simulink model "IEEE14_case"  (R2024b)
settings: Solver=FixedStepAuto  StartTime=0  StopTime=2  FixedStep=1e-7  RelTol=1e-3
values from neighbouring files (symbols this model uses):
  GFL_15_Bva = 0.009    [IEEE14_parameters.m]
  GFL_15_C_bus_pu = 7.179419    [IEEE14_parameters.m]
  GFL_15_f0 = 60    [IEEE14_parameters.m]
  GFL_15_I_id = 691.26967    [IEEE14_parameters.m]
  GFL_15_I_iq = 691.26967    [IEEE14_parameters.m]
  GFL_15_I_od = 45.2207    [IEEE14_parameters.m]
  GFL_15_I_oq = 45.2207    [IEEE14_parameters.m]
  GFL_15_I_pll = 0.78    [IEEE14_parameters.m]
  GFL_15_Kdi = 0.09    [IEEE14_parameters.m]
  GFL_15_Kdo = 0.9    [IEEE14_parameters.m]
  GFL_15_Kqi = 0.09    [IEEE14_parameters.m]
  GFL_15_Kqo = 0.9    [IEEE14_parameters.m]
  GFL_15_Lg_pu = 0.631447    [IEEE14_parameters.m]
  GFL_15_mode = 1    [IEEE14_parameters.m]
  GFL_15_P_id = 3.7166    [IEEE14_parameters.m]
  GFL_15_P_iq = 3.7166    [IEEE14_parameters.m]
  GFL_15_P_od = 0.4798    [IEEE14_parameters.m]
  GFL_15_P_oq = 0.4798    [IEEE14_parameters.m]
  GFL_15_P_pll = 290.42    [IEEE14_parameters.m]
  GFL_15_Qe_ref = 0.2    [IEEE14_parameters.m]
  GFL_15_Rg_pu = 0.024016    [IEEE14_parameters.m]
  GFL_15_Sbase = 1.000000e+4    (= 10000)    [IEEE14_parameters.m]
  GFL_15_Tdi = 0.01    [IEEE14_parameters.m]
  GFL_15_Tdo = 0.2    [IEEE14_parameters.m]
  GFL_15_Tqi = 0.01    [IEEE14_parameters.m]
  GFL_15_Tqo = 0.2    [IEEE14_parameters.m]
  GFL_15_Vbase = 380    [IEEE14_parameters.m]
  GFL_15_Vdc_ref = 1.011475    [IEEE14_parameters.m]
  GFL_15_Vdcbase = 700    [IEEE14_parameters.m]
  GFL_15_vq_ref = 0    [IEEE14_parameters.m]
  GFL_16_Bva = 0.002    [IEEE14_parameters.m]
  GFL_16_C_bus_pu = 7.179419    [IEEE14_parameters.m]
  GFL_16_f0 = 60    [IEEE14_parameters.m]
  GFL_16_I_id = 691.26967    [IEEE14_parameters.m]
  GFL_16_I_iq = 691.26967    [IEEE14_parameters.m]
  GFL_16_I_od = 45.2207    [IEEE14_parameters.m]
  GFL_16_I_oq = 45.2207    [IEEE14_parameters.m]
  GFL_16_I_pll = 0.78    [IEEE14_parameters.m]
  GFL_16_Kdi = 0.05    [IEEE14_parameters.m]
  GFL_16_Kdo = 0.5    [IEEE14_parameters.m]
  GFL_16_Kqi = 0.05    [IEEE14_parameters.m]
  GFL_16_Kqo = 0.5    [IEEE14_parameters.m]
  GFL_16_Lg_pu = 0.631447    [IEEE14_parameters.m]
  GFL_16_mode = 1    [IEEE14_parameters.m]
  GFL_16_P_id = 3.7166    [IEEE14_parameters.m]
  GFL_16_P_iq = 3.7166    [IEEE14_parameters.m]
  GFL_16_P_od = 0.4798    [IEEE14_parameters.m]
  GFL_16_P_oq = 0.4798    [IEEE14_parameters.m]
  GFL_16_P_pll = 290.42    [IEEE14_parameters.m]
  GFL_16_Qe_ref = 0.2    [IEEE14_parameters.m]
  GFL_16_Rg_pu = 0.024016    [IEEE14_parameters.m]
  GFL_16_Sbase = 1.000000e+4    (= 10000)    [IEEE14_parameters.m]
  GFL_16_Tdi = 0.01    [IEEE14_parameters.m]
  GFL_16_Tdo = 0.2    [IEEE14_parameters.m]
  GFL_16_Tqi = 0.01    [IEEE14_parameters.m]
  GFL_16_Tqo = 0.2    [IEEE14_parameters.m]
  GFL_16_Vbase = 380    [IEEE14_parameters.m]
  GFL_16_Vdc_ref = 1.01144    [IEEE14_parameters.m]
  GFL_16_Vdcbase = 700    [IEEE14_parameters.m]
  GFL_16_vq_ref = 0    [IEEE14_parameters.m]
  GFL_17_Bva = 0.002    [IEEE14_parameters.m]
  GFL_17_C_bus_pu = 7.179419    [IEEE14_parameters.m]
  GFL_17_f0 = 60    [IEEE14_parameters.m]
  GFL_17_I_id = 691.26967    [IEEE14_parameters.m]
  GFL_17_I_iq = 691.26967    [IEEE14_parameters.m]
  GFL_17_I_od = 45.2207    [IEEE14_parameters.m]
  GFL_17_I_oq = 45.2207    [IEEE14_parameters.m]
  GFL_17_I_pll = 0.78    [IEEE14_parameters.m]
  GFL_17_Kdi = 0.05    [IEEE14_parameters.m]
  GFL_17_Kdo = 0.5    [IEEE14_parameters.m]
  GFL_17_Kqi = 0.05    [IEEE14_parameters.m]
  GFL_17_Kqo = 0.5    [IEEE14_parameters.m]
  GFL_17_Lg_pu = 0.631447    [IEEE14_parameters.m]
  GFL_17_mode = 1    [IEEE14_parameters.m]
  GFL_17_P_id = 3.7166    [IEEE14_parameters.m]
  GFL_17_P_iq = 3.7166    [IEEE14_parameters.m]
  GFL_17_P_od = 0.4798    [IEEE14_parameters.m]
  GFL_17_P_oq = 0.4798    [IEEE14_parameters.m]
  GFL_17_P_pll = 290.42    [IEEE14_parameters.m]
  GFL_17_Qe_ref = 0.2    [IEEE14_parameters.m]
  GFL_17_Rg_pu = 0.024016    [IEEE14_parameters.m]
  GFL_17_Sbase = 1.000000e+4    (= 10000)    [IEEE14_parameters.m]
  GFL_17_Tdi = 0.01    [IEEE14_parameters.m]
  GFL_17_Tdo = 0.2    [IEEE14_parameters.m]
  GFL_17_Tqi = 0.01    [IEEE14_parameters.m]
  GFL_17_Tqo = 0.2    [IEEE14_parameters.m]
  GFL_17_Vbase = 380    [IEEE14_parameters.m]
  GFL_17_Vdc_ref = 1.011632    [IEEE14_parameters.m]
  GFL_17_Vdcbase = 700    [IEEE14_parameters.m]
  GFL_17_vq_ref = 0    [IEEE14_parameters.m]
  GFL_18_Bva = 0.002    [IEEE14_parameters.m]
  GFL_18_C_bus_pu = 7.179419    [IEEE14_parameters.m]
  GFL_18_f0 = 60    [IEEE14_parameters.m]
  GFL_18_I_id = 691.26967    [IEEE14_parameters.m]
  GFL_18_I_iq = 691.26967    [IEEE14_parameters.m]
  GFL_18_I_od = 45.2207    [IEEE14_parameters.m]
  GFL_18_I_oq = 45.2207    [IEEE14_parameters.m]
  GFL_18_I_pll = 0.78    [IEEE14_parameters.m]
  GFL_18_Kdi = 0.05    [IEEE14_parameters.m]
  GFL_18_Kdo = 0.5    [IEEE14_parameters.m]
  GFL_18_Kqi = 0.05    [IEEE14_parameters.m]
  GFL_18_Kqo = 0.5    [IEEE14_parameters.m]
  GFL_18_Lg_pu = 0.631447    [IEEE14_parameters.m]
  GFL_18_mode = 1    [IEEE14_parameters.m]
  GFL_18_P_id = 3.7166    [IEEE14_parameters.m]
  GFL_18_P_iq = 3.7166    [IEEE14_parameters.m]
  GFL_18_P_od = 0.4798    [IEEE14_parameters.m]
  GFL_18_P_oq = 0.4798    [IEEE14_parameters.m]
  GFL_18_P_pll = 290.42    [IEEE14_parameters.m]
  GFL_18_Qe_ref = 0.2    [IEEE14_parameters.m]
  GFL_18_Rg_pu = 0.024016    [IEEE14_parameters.m]
  GFL_18_Sbase = 1.000000e+4    (= 10000)    [IEEE14_parameters.m]
  GFL_18_Tdi = 0.01    [IEEE14_parameters.m]
  GFL_18_Tdo = 0.2    [IEEE14_parameters.m]
  GFL_18_Tqi = 0.01    [IEEE14_parameters.m]
  GFL_18_Tqo = 0.2    [IEEE14_parameters.m]
  GFL_18_Vbase = 380    [IEEE14_parameters.m]
  GFL_18_Vdc_ref = 1.011572    [IEEE14_parameters.m]
  GFL_18_Vdcbase = 700    [IEEE14_parameters.m]
  GFL_18_vq_ref = 0    [IEEE14_parameters.m]
  ... (+180 more)
(part 25 of 25)

== system IEEE14_case/SG_D_8/i_q_SG_D_8_block ==
  note: i_q_SG_D_8 in case14gfl
      | $-\frac{\sin\left(\theta _{\mathrm{SG},D,8}\right)\,\left(\psi _{q,\mathrm{SG},D,8}+\frac{\psi _{\mathrm{gq},\mathrm{SG},D,8}\,\left(x_{l}-x_{\mathrm{qdd}}\right)}{x_{l}-x_{\mathrm{qd}}}+\frac{\psi _{\mathrm{kq},\mathrm{SG},D,8}\,\left(x_{\mathrm{qd}}-x_{\mathrm{qdd}}\right)}{x_{l}-x_{\mathrm{qd}}}\right)}{x_{\mathrm{qdd}}}-\frac{\cos\left(\theta _{\mathrm{SG},D,8}\right)\,\left(\frac{\psi _{\mathrm{1d},\mathrm{SG},D,8}\,\left(x_{\mathrm{dd}}-x_{\mathrm{ddd}}\right)}{x_{\mathrm{dd}}-x_{l}}-\psi _{d,\mathrm{SG},D,8}+\frac{\psi _{\mathrm{fd},\mathrm{SG},D,8}\,\left(x_{\mathrm{ddd}}-x_{l}\right)}{x_{\mathrm{dd}}-x_{l}}\right)}{x_{\mathrm{ddd}}}$
      | Automatically generated on 2025-10-09 21:34:36 .
  State_psi_gq_SG_D_8_d57d0 : Inport
  State_psi_kq_SG_D_8_4aaa9 : Inport  Port=2
  State_psi_q_SG_D_8_a812b : Inport  Port=3
  State_theta_SG_D_8_df609 : Inport  Port=4
  State_psi_1d_SG_D_8_47e6f : Inport  Port=5
  State_psi_d_SG_D_8_17299 : Inport  Port=6
  State_psi_fd_SG_D_8_e7c26 : Inport  Port=7
  State_theta_SG_D_8_83255 : Inport  Port=8
  Add_0afba : Sum
  Add_674ef : Sum
  Add_7283f : Sum
  Add_a0d89 : Sum
  Add_aa088 : Sum
  Add_f38dc : Sum
  Constant_-1_0e725 : Constant  Value=-1
  Constant_-1_483b1 : Constant  Value=-1
  Constant_-1_6ec14 : Constant  Value=-1
  Constant_-1_73685 : Constant  Value=-1
  Constant_-1_882c9 : Constant  Value=-1
  Constant_x_dd_3705f : Constant  Value=x_dd
  Constant_x_dd_b1fed : Constant  Value=x_dd
  Constant_x_dd_ff658 : Constant  Value=x_dd
  Constant_x_ddd_9f145 : Constant  Value=x_ddd
  Constant_x_ddd_c8c7b : Constant  Value=x_ddd
  Constant_x_ddd_d0b75 : Constant  Value=x_ddd
  Constant_x_l_4334d : Constant  Value=x_l
  Constant_x_l_5789b : Constant  Value=x_l
  Constant_x_l_6da42 : Constant  Value=x_l
  Constant_x_l_9a561 : Constant  Value=x_l
  Constant_x_l_9ddb0 : Constant  Value=x_l
  Constant_x_l_cc5c0 : Constant  Value=x_l
  Constant_x_qd_4d435 : Constant  Value=x_qd
  Constant_x_qd_6b128 : Constant  Value=x_qd
  Constant_x_qd_d2cb1 : Constant  Value=x_qd
  Constant_x_qdd_13df1 : Constant  Value=x_qdd
  Constant_x_qdd_6e527 : Constant  Value=x_qdd
  Constant_x_qdd_80335 : Constant  Value=x_qdd
  Divide_169a7 : Product  Inputs=*/
  Divide_2d472 : Product  Inputs=*/
  Divide_6c1fd : Product  Inputs=*/
  Divide_95db2 : Product  Inputs=*/
  Divide_c120f : Product  Inputs=*/
  Divide_c759c : Product  Inputs=*/
  MathFunc_cos_2d5cc : Trigonometry  Operator=cos
  MathFunc_sin_ab68c : Trigonometry
  Product_4d046 : Product
  Product_5b6e1 : Product
  Product_7cbb0 : Product
  Product_91f0e : Product
  Product_930c1 : Product
  Product_94d00 : Product
  Product_baa3a : Product
  Product_cba92 : Product
  Product_da788 : Product
  Product_f969b : Product
  Product_fd765 : Product
  Subtract_0cf3e : Sum  Inputs=+-
  Subtract_176ca : Sum  Inputs=+-
  Subtract_23062 : Sum  Inputs=+-
  Subtract_734e3 : Sum  Inputs=+-
  Subtract_af5a2 : Sum  Inputs=+-
  Subtract_c032e : Sum  Inputs=+-
  Subtract_f88e6 : Sum  Inputs=+-
  Blockout_i_q_SG_D_8_09699 : Outport
  wires:
  Constant_x_l_5789b/1 -> Product_5b6e1/2
  Constant_-1_483b1/1 -> Product_5b6e1/1
  Product_5b6e1/1 -> Add_0afba/1
  Product_930c1/1 -> Product_4d046/1
  Constant_-1_882c9/1 -> Product_930c1/1
  Constant_x_qdd_80335/1 -> Subtract_0cf3e/2
  Constant_x_qdd_6e527/1 -> Add_0afba/2
  Constant_x_qdd_13df1/1 -> Divide_6c1fd/2
  Product_f969b/1 -> Add_aa088/1
  Constant_-1_6ec14/1 -> Product_f969b/1
  Constant_x_l_4334d/1 -> Product_f969b/2
  Subtract_0cf3e/1 -> Product_cba92/2
  Constant_x_qd_d2cb1/1 -> Subtract_0cf3e/1
  Product_94d00/1 -> Divide_c120f/1
  Product_7cbb0/1 -> Add_f38dc/1
  Constant_-1_73685/1 -> Product_7cbb0/1
  Subtract_af5a2/1 -> Product_da788/1
  Constant_x_l_cc5c0/1 -> Product_7cbb0/2
  State_psi_1d_SG_D_8_47e6f/1 -> Product_930c1/2
  State_psi_gq_SG_D_8_d57d0/1 -> Product_94d00/1
  Add_0afba/1 -> Product_94d00/2
  MathFunc_sin_ab68c/1 -> Product_91f0e/2
  Constant_x_qd_4d435/1 -> Add_aa088/2
  Product_cba92/1 -> Divide_169a7/1
  State_psi_kq_SG_D_8_4aaa9/1 -> Product_cba92/1
  Add_7283f/1 -> Subtract_af5a2/1
  Constant_x_qd_6b128/1 -> Add_f38dc/2
  Subtract_176ca/1 -> Product_4d046/2
  Constant_x_dd_b1fed/1 -> Subtract_176ca/1
  Constant_x_ddd_d0b75/1 -> Subtract_176ca/2
  Add_aa088/1 -> Divide_c120f/2
  Add_f38dc/1 -> Divide_169a7/2
  Constant_-1_0e725/1 -> Product_fd765/1
  Subtract_23062/1 -> Divide_2d472/2
  Constant_x_dd_3705f/1 -> Subtract_23062/1
  Constant_x_l_9ddb0/1 -> Subtract_23062/2
  Add_a0d89/1 -> Product_fd765/2
  Subtract_734e3/1 -> Product_baa3a/2
  Constant_x_ddd_c8c7b/1 -> Subtract_734e3/1
  Constant_x_l_6da42/1 -> Subtract_734e3/2
  Constant_x_l_9a561/1 -> Subtract_f88e6/2
  Divide_c120f/1 -> Subtract_c032e/1
  State_psi_q_SG_D_8_a812b/1 -> Add_a0d89/2
  Divide_169a7/1 -> Subtract_c032e/2
  Product_4d046/1 -> Divide_2d472/1
  Constant_x_ddd_9f145/1 -> Divide_95db2/2
  Product_baa3a/1 -> Divide_c759c/1
  State_psi_fd_SG_D_8_e7c26/1 -> Product_baa3a/1
  Subtract_f88e6/1 -> Divide_c759c/2
  Constant_x_dd_ff658/1 -> Subtract_f88e6/1
  Subtract_c032e/1 -> Add_a0d89/1
  Divide_2d472/1 -> Add_7283f/1
  State_psi_d_SG_D_8_17299/1 -> Add_7283f/2
  State_theta_SG_D_8_df609/1 -> MathFunc_sin_ab68c/1
  Product_91f0e/1 -> Divide_6c1fd/1
  Divide_c759c/1 -> Subtract_af5a2/2
  MathFunc_cos_2d5cc/1 -> Product_da788/2
  State_theta_SG_D_8_83255/1 -> MathFunc_cos_2d5cc/1
  Product_fd765/1 -> Product_91f0e/1
  Product_da788/1 -> Divide_95db2/1
  Divide_6c1fd/1 -> Add_674ef/1
  Add_674ef/1 -> Blockout_i_q_SG_D_8_09699/1
  Divide_95db2/1 -> Add_674ef/2

== system IEEE14_case/SG_D_8/theta_SG_D_8_out_block ==
  note: theta_SG_D_8_out in case14gfl
      | $\theta _{\mathrm{SG},D,8}$
      | Automatically generated on 2025-10-09 21:34:41 .
  State_theta_SG_D_8_cdb63 : Inport
  Blockout_theta_SG_D_8_out_2e6e5 : Outport
  wires:
  State_theta_SG_D_8_cdb63/1 -> Blockout_theta_SG_D_8_out_2e6e5/1

== system IEEE14_case/SG_D_8/w_SG_D_8_out_block ==
  note: w_SG_D_8_out in case14gfl
      | $w_{\mathrm{SG},D,8}$
      | Automatically generated on 2025-10-09 21:34:40 .
  State_w_SG_D_8_62717 : Inport
  Blockout_w_SG_D_8_out_d72e6 : Outport
  wires:
  State_w_SG_D_8_62717/1 -> Blockout_w_SG_D_8_out_d72e6/1
